simulink model "constraints_comparison_A_4D_v2"  (R2016a)
settings: Solver=ode4  StartTime=0.0  StopTime=total_time  FixedStep=0.0001  RelTol=1e-3
InitFcn:
  | % clear
  | % clc
undefined symbols (not defined in the file or in its folder): acm_aero_model, acm_T_N, breakpoints1, Cm0, Cmde, Cmq, comp_feedback, constraint_type, dail, de, dele, dele_trim, drud, Fr_mp_1, Fr_mp_2, Fr_rp_1, Fr_rp_2, ini_acm_de_deg, ini_acm_p_deg_per_s, ini_acm_phi_deg, ini_acm_psi_deg, ini_acm_q_deg_per_s, ini_acm_r_deg_per_s, ini_acm_theta_deg, ini_cmp_de_deg, ini_rig_p_deg_per_s, ini_rig_phi_deg, ini_rig_psi_deg, ini_rig_q_deg_per_s, ini_rig_r_deg_per_s, ini_rig_theta_deg, input_type, K1_svo_acm, K1_svo_cmp, K2_svo_acm, K2_svo_cmp, La, Ma, max_defl_sat_acm, max_defl_sat_cmp, max_rate_sat, max_rate_sat_acm, max_rate_sat_cmp, Na, radius, sigbuilder_block, simstop, theta_trim, thrust_trim, windspeed, Xa, Ya, Za
libraries: aerolibconvert2 x119, simulink x42, aerolibtransform2 x19, vrlib x2
(part 1 of 6)
settings Model: Creator=PD Banneheka  LastModifiedBy=PD Banneheka
settings DataIOCC: LimitDataPoints=on  SaveFormat=Array  SaveOutput=off  SaveTime=off
settings HardwareCC: ProdBitPerPointer=32  ProdLargestAtomicFloat=None  ProdIntDivRoundTo=Undefined  ProdEndianess=Unspecified  ProdWordSize=32  ProdHWDeviceType=32-bit Generic
settings ModelReferenceCC: PropagateSignalLabelsOutOfModel=off
settings ConfigComp: CovModelRefEnable=Off

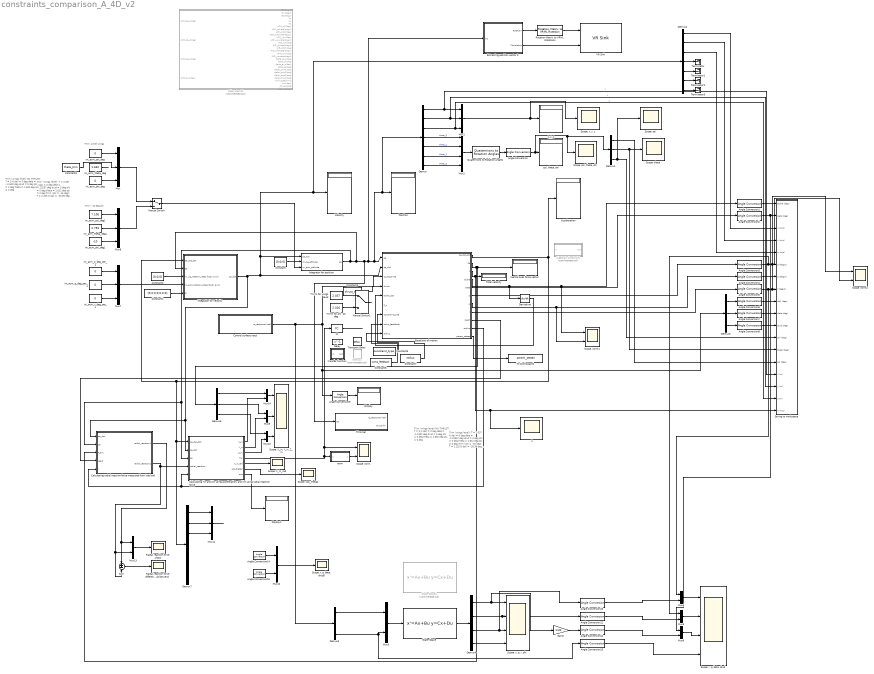
== system constraints_comparison_A_4D_v2 ==
  note: Trim: Level wings
  note: Trim (wings level):
      | T = 2.037 N
      | dail = 0 deg
      | dele = -1.22537 deg
      | drud = 0 deg
      | phi = 0 deg
      | theta = 1.612 deg
      | psi = 0 deg
      |
      | Trim (phi = -15 deg):
      | T = 2.225 N
      | dail = -30.39 deg
      | dele = -1.382 deg
      | drud = -36.89 deg
      | phi = -15.01 deg
      | theta = 5.134 deg
      | psi = 11.95 deg
      |
      | Trim (phi = -10 deg):
      | T = 2.026 N
      | dail = -18.93 deg
      | dele = -1.148 deg
      | drud = -22.97 deg
      | phi = -10 deg
      | theta = 2.793 deg
      | psi = 7.106 deg
  note: Trim (wings level):
      | T = 2.037 N
      | dail = 0 deg
      | dele = -1.22537 deg
      | drud = 0 deg
      | phi = 0 deg
      | theta = 1.612 deg
      | psi = 0 deg
      |
      | Trim (phi = -15 deg):
      | T = 2.225 N
      | dail = -30.39 deg
      | dele = -1.382 deg
      | drud = -36.89 deg
      | phi = -15.01 deg
      | theta = 5.134 deg
      | psi = 11.95 deg
      |
      | Trim (phi = -10 deg):
      | T = 2.026 N
      | dail = -18.93 deg
      | dele = -1.148 deg
      | drud = -22.97 deg
      | phi = -10 deg
      | theta = 2.793 deg
      | psi = 7.106 deg
  note: Trim: -10 deg phi
  note: Trim (wings level)
      | NO THRUST:
      | T = 0 N
      | dail = 0 deg
      | dele = -1.2402 deg
      | drud = 0 deg
      | phi = 0 deg
      | theta = 1.632 deg
      | psi = 0 deg
  note: Trim (wings level)
      | NO THRUST:
      | T = 0 N
      | dail = 0 deg
      | dele = -1.2402 deg
      | drud = 0 deg
      | phi = 0 deg
      | theta = 1.632 deg
      | psi = 0 deg
  Acceleration : Display
  Algebraic Constraint : Subsystem  Commented=on
  Angle Conversion{,1..15} (16 alike) : aerolibconvert2/Angle Conversion  IU=rad  OU=deg
  "Calculating Yin and Zin using acceleration, and Xin using radial reaction force" : MATLAB Function  TreatAsAtomicUnit=on
      settings: MinAlgLoopOccurrences=on
  Calculating radial reaction force measured from load cell : MATLAB Function  TreatAsAtomicUnit=on
      settings: MinAlgLoopOccurrences=on
  Constant : Constant  Value=[0;0;0]
  Constant1 : Constant  Value=[0;0;0;0;0;0;0]
  Constant2 : Constant  Value=[0;0;0]
  Constant3 : Constant  Value=theta_trim
  Constant4 : Constant  Value=thrust_trim
  Constant5 : Constant  Value=constraint_type
  Constant6 : Constant  Value=comp_feedback
  Constant7 : Constant  Value=radius
  Control surface input : Subsystem
  Delay : Delay  DelayLength=1  InitialCondition=0
  Demux : Demux  Outputs=7
  Demux{1,3,5..6} (4 alike) : Demux  Outputs=3
  Demux2 : Demux  Outputs=7
  Demux4 : Demux
  Demux7 : Demux  Outputs=7
  Derivative : Derivative
  Display : Display
  Display1 : Display
  Equations of motion : MATLAB Function  TreatAsAtomicUnit=on
      settings: MinAlgLoopOccurrences=on
  Extracting position vector 3 : Subsystem
  Gain2 : Gain  Gain=1/30
  IC : InitialCondition  Value=0
  Inertial axes force vector : Display
  Integrator for position : Subsystem  TreatAsAtomicUnit=on
      settings: MinAlgLoopOccurrences=on
  Integrator for velocity : Subsystem  TreatAsAtomicUnit=on
      settings: MinAlgLoopOccurrences=on
  Manual Switch : ManualSwitch
  Manual Switch1 : ManualSwitch
  Memory : Memory  Commented=on
  Mux{,1,7..8,11} (5 alike) : Mux  Inputs=3
  Mux{3..6,9..10,12..14} (9 alike) : Mux  Inputs=2
  Mux2 : Mux
  Position : Display
  Quaternions to Rotation Angles : aerolibtransform2/Quaternions to Rotation Angles  rotationOrder=ZYX
  Radial reaction force check : Scope
  Radial reaction force difference (should be zero) : Scope
  Rotation Matrix to VRML Rotation4 : vrlib/Utilities/Rotation Matrix to VRML Rotation  maxzero=1e-12
  Saving to workspace : Subsystem
  "Scope: X_in, Y_in, Z_in" : Scope  NumInputPorts=3
  Scope: X_in_rad : Scope
  Scope: cos_theta2 : Scope
  Scope: norm : Scope  NumInputPorts=2
  Scope: norm1 : Scope  NumInputPorts=2
  Scope: norm2 : Scope  NumInputPorts=2
  Scope: psi : Scope
  "Scope: psi, theta, phi" : Scope
  "Scope: r, p, beta, drud" : Scope  NumInputPorts=4
  "Scope: r, p, beta, drud5" : Scope
  Scope: theta : Scope
  "Scope: v, p, r, phi" : Scope  NumInputPorts=4
  "Scope: x, y, z" : Scope
  State-Space : StateSpace  A="[-0.8650         0  -30.0000    9.8100; -9.3510   -5.8803    2.8245         0; 5.4903   -0.1244   -2.0599         0; 0    1.0000         0         0]"  B="[0    4.5016; -213.0227  266.8872; -52.0114  -10.7994; 0         0]"  C=[1 0 0 0; 0 1 0 0; 0 0 1 0; 0 0 0 1]  D=[0 0; 0 0; 0 0; 0 0]  X0=0
  State-Space1 : StateSpace  Commented=on  A="[-0.8650         0         -30    9.8100; -10.2332   -5.8603    3.1556         0; 5.9066    0.1374   -2.1857         0; 0    1.0000         0         0]"  B="[0    4.5016; 204.6649 -268.6226; 42.5275   22.6814; 0         0]"  C=[1 0 0 0; 0 1 0 0; 0 0 1 0; 0 0 0 1]  D=[0 0; 0 0; 0 0; 0 0]  X0=0
  Subsystem14 : Subsystem  Commented=on
  Sum : Sum  Inputs=+-
  T trim for phi -10 deg : Constant  Value=2.026
  T trim for wings level : Constant  Value=2.037
  Terminator{,1..3} (4 alike) : Terminator
  To Workspace1 : ToWorkspace  VariableName=param_states  SaveFormat=Timeseries  SampleTime=-1
  Total velocity : Display
  Transport Delay : TransportDelay  DelayTime=0.1
  Trimmer : Subsystem
  V : Scope
  VR Sink : vrlib/VR Sink  InstantiateOnLoad=on  SampleTime=-1  ViewEnable=on  RemoteChange=off  RemoteView=off  FieldsWritten=Aircraft_model.rotation.4.1.1.double#Aircraft_model.translation.3.1.1.double  WorldFileName=Animation.wrl  AutoView=on  VideoDimensions=[]  AllowVariableSize=off  FigureProperties="{'Position', 'Name', 'Viewpoint', 'CameraBound', 'CameraDirection', 'CameraPosition', 'CameraUpVector', 'ZoomFactor', 'Antialiasing', 'Headlight', 'Lighting', 'NavPanel', 'Sound', 'StatusBar', 'Stereo3D', 'Stereo3DCameraOffset', 'Stereo3DHIT', 'ToolBar', 'Textures', 'Transparency', 'Triad', 'Wireframe', 'NavZones', 'NavMode', 'NavSpeed', 'CaptureFileFormat', 'CaptureFileName', 'Record2DCompressMethod', 'Record2DCompressQuality', 'Record2D', 'Record2DFileName', 'Record2DFPS'; [5.0000000000000000e+00   9.2000000000000000e+01   5.7600000000000000e+02   3.5000000000000000e+02], '', 'Front view', 'on', [0.0000000000000000e+00   0.0000000000000000e+00  -1.0000000000000000e+00], [0.0000000000000000e+00   0.0000000000000000e+00   0.0000000000000000e+00], [0.0000000000000000e+00   1.0000000000000000e+00   0.0000000000000000e+00], [1.0000000000000000e+00], 'on', 'on', 'on', 'halfbar', 'on', 'on', 'off', [1.0000000149011612e-01], [0.0000000000000000e+00], 'on', 'on', 'on', 'none', 'off', 'off', 'fly', 'normal', 'tif', '%f_anim_%n.tif', 'auto', [7.5000000000000000e+01], 'off', '%f_anim_%n.avi', 'auto'}"
  Velocity : Display
  ini_acm_p_deg_per_s : Constant  Value=0
  ini_acm_phi_deg : Constant  Value=0
  ini_acm_phi_deg1 : Constant  Value=-10
  ini_acm_psi_deg : Constant  Value=0
  ini_acm_psi_deg1 : Constant  Value=7.106
  ini_acm_q_deg_per_s : Constant  Value=0
  ini_acm_r_deg_per_s : Constant  Value=0
  ini_acm_theta_deg : Constant  Value=1.632
  ini_acm_theta_deg1 : Constant  Value=2.793
  norm : MATLAB Function  TreatAsAtomicUnit=on
  "psi, theta, phi" : Display
  transfer function : Subsystem  TreatAsAtomicUnit=on
      settings: MinAlgLoopOccurrences=on
  "x, y, z" : Display
  wires:
  Manual Switch/1 -> Integrator for position/3(ini_acm_attitude)
  Mux7/1 -> Integrator for velocity/4(ini_acm_rotation_rates (body axis))
  ini_acm_psi_deg/1 -> Mux/1
  ini_acm_theta_deg/1 -> ?
  ini_acm_phi_deg/1 -> Mux/3
  ini_acm_p_deg_per_s/1 -> Mux7/1
  ini_acm_r_deg_per_s/1 -> Mux7/3
  ini_acm_q_deg_per_s/1 -> Mux7/2
  Integrator for velocity/1(qa_dot) -> Calculating radial reaction force measured from load cell/1(qa_dot), "Calculating Yin and Zin using acceleration, and Xin using radial reaction force"/2(qa_dot), Demux2/1, Velocity/1, Integrator for position/1(qa_dot), Equations of motion/2(qa_dot)
  Constant/1 -> Integrator for position/2(ini_rig_attitude)
  Constant1/1 -> Integrator for velocity/5(qr)
  Constant2/1 -> Integrator for velocity/3(ini_rig_rotation_rates (body axis))
  Demux/4 -> Mux2/1  "theta_0"
  Demux/5 -> Mux2/2  "theta_1"
  Demux/6 -> Mux2/3  "theta_2"
  Demux/7 -> Mux2/4  "theta_3"
  Demux/3 -> Saving to workspace/17(z (m)), Mux1/3  "z"
  Demux/2 -> Saving to workspace/16(y (m)), Mux1/2  "y"
  Demux/1 -> Saving to workspace/15(x (m)), Mux1/1  "x"
  Mux1/1 -> "Scope: x, y, z"/1, "x, y, z"/1
  Mux2/1 -> Quaternions to Rotation Angles/1
  Quaternions to Rotation Angles/1 -> Angle Conversion/1
  Angle Conversion/1 -> Demux1/1, "Scope: psi, theta, phi"/1, "psi, theta, phi"/1
  Equations of motion/2(Fa) -> Demux6/1, Inertial axes force vector/1, Calculating radial reaction force measured from load cell/3(F_ext)
  Equations of motion/3(V) -> V/1, Saving to workspace/18(V (m/s)), Total velocity/1
  Equations of motion/1(qa_dot_dot) -> Integrator for velocity/1(qa_dot_dot), Demux7/1, "Calculating Yin and Zin using acceleration, and Xin using radial reaction force"/1(qa_dot_dot), Acceleration/1
  Equations of motion/4(alpha) -> Derivative/1, Scope: norm1/1, Angle Conversion1/1
  Integrator for position/1(qa) -> "Calculating Yin and Zin using acceleration, and Xin using radial reaction force"/3(qa), Calculating radial reaction force measured from load cell/2(qa), Integrator for velocity/2(qa), Trimmer/1(qa), Extracting position vector 3/1(In1), Demux/1, Position/1, Equations of motion/1(qa)
  Extracting position vector 3/1(Rotation) -> Rotation Matrix to VRML Rotation4/1
  Extracting position vector 3/2(Translation) -> VR Sink/2
  Rotation Matrix to VRML Rotation4/1 -> VR Sink/1
  Manual Switch1/1 -> ?
  Angle Conversion1/1 -> Saving to workspace/1(alpha (deg))
  Equations of motion/5(beta) -> Angle Conversion2/1
  Demux2/4 -> Terminator/1
  Demux2/6 -> Terminator2/1
  Demux2/7 -> Terminator3/1
  Demux2/5 -> Terminator1/1
  Demux2/1 -> Saving to workspace/3(u (m/s))
  Demux2/2 -> Saving to workspace/4(v (m/s))
  Demux2/3 -> Saving to workspace/5(w (m/s))
  Angle Conversion3/1 -> Mux5/1, Scope: norm2/2, Saving to workspace/6(p (deg/s))
  Angle Conversion5/1 -> Mux4/1, Scope: norm2/1, Saving to workspace/8(r (deg/s))
  Angle Conversion4/1 -> Saving to workspace/7(q (deg/s))
  Equations of motion/6(p) -> Angle Conversion3/1
  Equations of motion/7(q) -> Scope: norm1/2, Angle Conversion4/1
  Equations of motion/8(r) -> Angle Conversion5/1
  Demux3/1 -> Angle Conversion6/1
  Demux3/2 -> Angle Conversion7/1
  Demux3/3 -> Angle Conversion8/1
  Control surface input/1(cs_response (rad)) -> Equations of motion/3(cs_response), Demux3/1, Angle Conversion9/1, Demux5/1
  Demux1/1 -> Saving to workspace/14(psi (deg))
  Demux1/2 -> Saving to workspace/13(theta (deg)), Scope: theta/1
  Demux1/3 -> Scope: psi/1, Saving to workspace/12(phi (deg))
  Angle Conversion6/1 -> Saving to workspace/9(dail (deg))
  Angle Conversion7/1 -> Saving to workspace/10(dele (deg))
  Angle Conversion8/1 -> Saving to workspace/11(drud (deg))
  Mux3/1 -> State-Space/1
  State-Space/1 -> Demux4/1
  Demux5/1 -> Mux3/1
  Demux5/3 -> Mux3/2, Angle Conversion13/1
  Demux4/1 -> Gain2/1, "Scope: v, p, r, phi"/1
  Demux4/2 -> Angle Conversion11/1, "Scope: v, p, r, phi"/2
  Demux4/3 -> Angle Conversion10/1, "Scope: v, p, r, phi"/3
  Demux4/4 -> "Scope: v, p, r, phi"/4
  Gain2/1 -> Angle Conversion12/1
  Angle Conversion10/1 -> Mux4/2
  Angle Conversion11/1 -> Mux5/2
  Angle Conversion12/1 -> Mux6/2
  Mux4/1 -> "Scope: r, p, beta, drud"/1
  Mux5/1 -> "Scope: r, p, beta, drud"/2
  Mux6/1 -> "Scope: r, p, beta, drud"/3
  Angle Conversion13/1 -> "Scope: r, p, beta, drud"/4
  Angle Conversion2/1 -> Mux6/1, Saving to workspace/2(beta (deg))
  Angle Conversion9/1 -> Display/1
  Mux/1 -> Manual Switch/1
  ini_acm_psi_deg1/1 -> Mux8/1
  ini_acm_theta_deg1/1 -> Mux8/2
  ini_acm_phi_deg1/1 -> Mux8/3
  Mux8/1 -> Manual Switch/2
  T trim for wings level/1 -> Manual Switch1/1
  T trim for phi -10 deg/1 -> Manual Switch1/2
  "Calculating Yin and Zin using acceleration, and Xin using radial reaction force"/3(Z_in) -> Mux10/2
  "Calculating Yin and Zin using acceleration, and Xin using radial reaction force"/2(Y_in) -> Mux9/2
  Demux6/2 -> Mux9/1
  Demux6/3 -> Mux10/1
  Mux9/1 -> "Scope: X_in, Y_in, Z_in"/2
  Mux10/1 -> "Scope: X_in, Y_in, Z_in"/3
  Demux7/3 -> Mux11/3
  Demux7/2 -> Mux11/2
  Demux7/1 -> Mux11/1
  Mux11/1 -> ?
  Angle Conversion14/1 -> Mux12/1
  Angle Conversion15/1 -> Mux12/2
  Mux12/1 -> "Scope: r, p, beta, drud5"/1
  Equations of motion/9(react) -> Calculating radial reaction force measured from load cell/4(react)
  Calculating radial reaction force measured from load cell/1(radial_reaction1) -> Sum/1, Mux13/1
  Calculating radial reaction force measured from load cell/2(radial_reaction2) -> Sum/2, Mux13/2, "Calculating Yin and Zin using acceleration, and Xin using radial reaction force"/4(radial_reaction)
  Mux13/1 -> Radial reaction force check/1
  Sum/1 -> Radial reaction force difference (should be zero)/1
  Mux14/1 -> "Scope: X_in, Y_in, Z_in"/1
  Demux6/1 -> Mux14/1
  "Calculating Yin and Zin using acceleration, and Xin using radial reaction force"/1(X_in) -> Mux14/2
  Equations of motion/10(radius) -> Calculating radial reaction force measured from load cell/5(r), "Calculating Yin and Zin using acceleration, and Xin using radial reaction force"/5(r)
  "Calculating Yin and Zin using acceleration, and Xin using radial reaction force"/5(X_in_rad) -> Scope: X_in_rad/1
  "Calculating Yin and Zin using acceleration, and Xin using radial reaction force"/6(cos_theta2) -> Scope: cos_theta2/1
  "Calculating Yin and Zin using acceleration, and Xin using radial reaction force"/7(pos) -> Display1/1
  "Calculating Yin and Zin using acceleration, and Xin using radial reaction force"/4(F_c) -> norm/1(u), IC/1, Scope: norm/1
  norm/1(y) -> Scope: norm/2
  Derivative/1 -> Equations of motion/5(alpha_dot)
  Equations of motion/11(param_states) -> To Workspace1/1
  Constant3/1 -> Mux/2
  Constant4/1 -> Equations of motion/4(thrust)
  Constant5/1 -> Equations of motion/7(constraint_type)
  Constant6/1 -> Equations of motion/8(comp_feedback)
  IC/1 -> ?
  Constant7/1 -> Equations of motion/9("radius ")

== system constraints_comparison_A_4D_v2/Algebraic Constraint ==
  In : Inport
  Algebraic Constraint : simulink/Math Operations/Algebraic Constraint  z0=0.05076
  Algebraic Constraint{1,3..6} (5 alike) : simulink/Math Operations/Algebraic Constraint  z0=0
  Algebraic Constraint2 : simulink/Math Operations/Algebraic Constraint  z0=-0.05076
  Demux : Demux  Outputs=7
  Mux : Mux  Inputs=7
  Out : Outport
  wires:
  In/1 -> Demux/1
  Demux/7 -> Algebraic Constraint6/1
  Demux/1 -> Algebraic Constraint/1
  Demux/2 -> Algebraic Constraint1/1
  Demux/3 -> Algebraic Constraint2/1
  Demux/4 -> Algebraic Constraint3/1
  Demux/5 -> Algebraic Constraint4/1
  Demux/6 -> Algebraic Constraint5/1
  Algebraic Constraint6/1 -> Mux/7
  Algebraic Constraint5/1 -> Mux/6
  Algebraic Constraint4/1 -> Mux/5
  Algebraic Constraint3/1 -> Mux/4
  Algebraic Constraint2/1 -> Mux/3
  Algebraic Constraint1/1 -> Mux/2
  Algebraic Constraint/1 -> Mux/1
  Mux/1 -> Out/1

== system constraints_comparison_A_4D_v2/Control surface input ==
  1) Short period : Subsystem
  2) Phugoid : Subsystem  Commented=on
  3) Roll subsidence : Subsystem
  4) Spiral : Subsystem
  5) Dutch roll : Subsystem
  Aileron servo transfer function : TransferFcn  Denominator=[0.0025 0.08 1]
  Constant1 : Constant  Value=input_type
  Constant5 : Constant  Value=5
  Demux : Demux  Outputs=3
  Elevator servo transfer function : TransferFcn  Denominator=[0.0025 0.08 1]
  Manual Switch : ManualSwitch  CurrentSetting=0
  Manual Switch1 : ManualSwitch  CurrentSetting=0
  Manual Switch2 : ManualSwitch  CurrentSetting=0
  Multiport Switch : MultiPortSwitch  Inputs=5
  Mux : Mux  Inputs=3
  Rudder servo transfer function : TransferFcn  Denominator=[0.0025 0.08 1]
  cs_response (rad) : Outport
  wires:
  Manual Switch2/1 -> Mux/3  "drud"
  Manual Switch/1 -> Mux/1  "dail"
  Mux/1 -> cs_response (rad)/1
  1) Short period/1(cs_command (rad)) -> Multiport Switch/2
  2) Phugoid/1(cs_command (rad)) -> Multiport Switch/3
  3) Roll subsidence/1(cs_command (rad)) -> Multiport Switch/4
  4) Spiral/1(cs_command (rad)) -> Multiport Switch/5
  5) Dutch roll/1(cs_command (rad)) -> Multiport Switch/6
  Constant5/1 -> ?
  Multiport Switch/1 -> Demux/1
  Demux/1 -> Manual Switch/2, Aileron servo transfer function/1
  Demux/2 -> Manual Switch1/2, Elevator servo transfer function/1
  Demux/3 -> Manual Switch2/2, Rudder servo transfer function/1
  Manual Switch1/1 -> Mux/2  "dele"
  Aileron servo transfer function/1 -> Manual Switch/1  "dail"
  Elevator servo transfer function/1 -> Manual Switch1/1  "dele"
  Rudder servo transfer function/1 -> Manual Switch2/1  "drud"
  Constant1/1 -> Multiport Switch/1

== system constraints_comparison_A_4D_v2/Extracting position vector 3 ==
  In1 : Inport
  MATLAB Function : MATLAB Function  TreatAsAtomicUnit=on
  MATLAB Function1 : MATLAB Function  TreatAsAtomicUnit=on
  MATLAB Function6 : MATLAB Function  TreatAsAtomicUnit=on
  Rotation : Outport
  Translation : Outport  Port=2
  wires:
  MATLAB Function/1(y) -> Translation/1
  In1/1 -> MATLAB Function1/1(qa), MATLAB Function/1(u)
  MATLAB Function1/1(Aa) -> MATLAB Function6/1(A3)
  MATLAB Function6/1(A33) -> Rotation/1

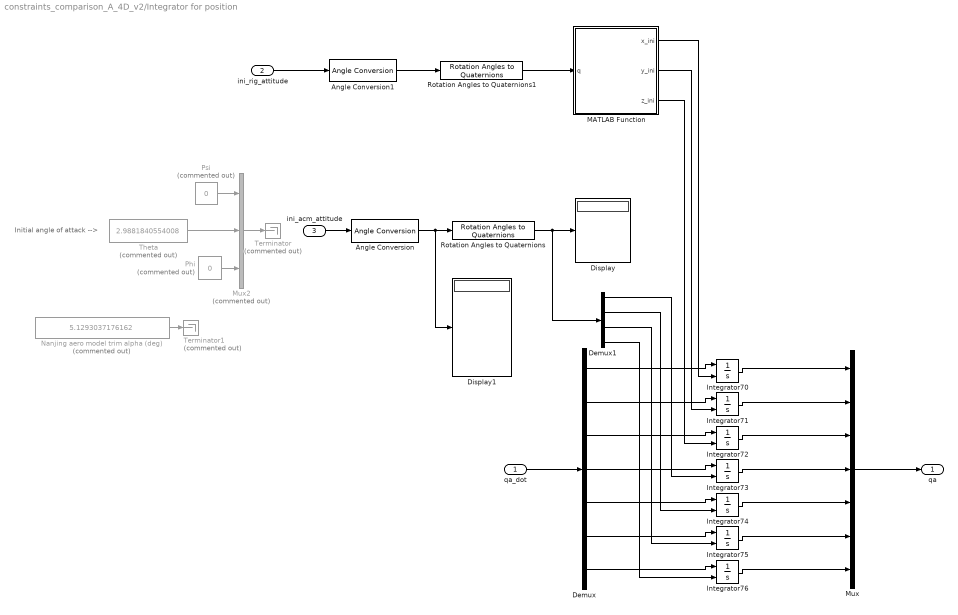
== system constraints_comparison_A_4D_v2/Integrator for position ==
  note: Initial angle of attack -->
  qa_dot : Inport
  ini_rig_attitude : Inport  Port=2
  ini_acm_attitude : Inport  Port=3
  Angle Conversion : aerolibconvert2/Angle Conversion  IU=deg  OU=rad
  Angle Conversion1 : aerolibconvert2/Angle Conversion  IU=deg  OU=rad
  Demux : Demux  Outputs=7
  Demux1 : Demux
  Display : Display
  Display1 : Display
  Integrator70 : Integrator  InitialConditionSource=external  InitialCondition=0.8
  Integrator{71..72,74..76} (5 alike) : Integrator  InitialConditionSource=external
  Integrator73 : Integrator  InitialConditionSource=external  InitialCondition=1
  MATLAB Function : MATLAB Function
  Mux : Mux  Inputs=7
  Mux2 : Mux  Commented=on  Inputs=3
  Nanjing aero model trim alpha (deg) : Constant  Commented=on  Value=5.1293037176162
  Phi : Constant  Commented=on  Value=0
  Psi : Constant  Commented=on  Value=0
  Rotation Angles to Quaternions : aerolibtransform2/Rotation Angles to Quaternions  rotationOrder=ZYX
  Rotation Angles to Quaternions1 : aerolibtransform2/Rotation Angles to Quaternions  rotationOrder=ZYX
  Terminator : Terminator  Commented=on
  Terminator1 : Terminator  Commented=on
  Theta : Constant  Commented=on  Value=2.9881840554008
  qa : Outport
  wires:
  Mux/1 -> qa/1
  qa_dot/1 -> Demux/1
  Demux/6 -> Integrator75/1
  Demux/5 -> Integrator74/1
  Demux/4 -> Integrator73/1
  Demux/3 -> Integrator72/1
  Demux/2 -> Integrator71/1
  Demux/7 -> Integrator76/1
  Demux/1 -> Integrator70/1
  Integrator76/1 -> Mux/7
  Integrator75/1 -> Mux/6
  Integrator74/1 -> Mux/5
  Integrator73/1 -> Mux/4
  Integrator72/1 -> Mux/3
  Integrator71/1 -> Mux/2
  Integrator70/1 -> Mux/1
  Phi/1 -> Mux2/3
  Psi/1 -> Mux2/1
  Mux2/1 -> Terminator/1
  Rotation Angles to Quaternions/1 -> Demux1/1, Display/1
  Demux1/4 -> Integrator76/2
  Demux1/1 -> Integrator73/2
  Demux1/2 -> Integrator74/2
  Demux1/3 -> Integrator75/2
  Angle Conversion/1 -> Display1/1, Rotation Angles to Quaternions/1
  Nanjing aero model trim alpha (deg)/1 -> Terminator1/1
  MATLAB Function/1(x_ini) -> Integrator70/2
  MATLAB Function/2(y_ini) -> Integrator71/2
  MATLAB Function/3(z_ini) -> Integrator72/2
  Theta/1 -> Mux2/2
  Angle Conversion1/1 -> Rotation Angles to Quaternions1/1
  ini_rig_attitude/1 -> Angle Conversion1/1
  ini_acm_attitude/1 -> Angle Conversion/1
  Rotation Angles to Quaternions1/1 -> MATLAB Function/1(q)

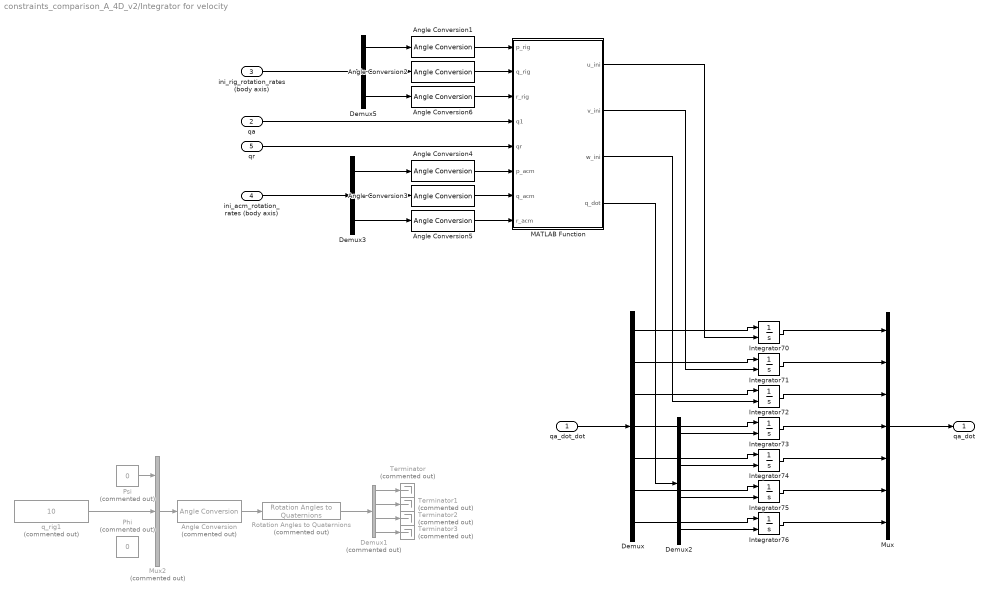
== system constraints_comparison_A_4D_v2/Integrator for velocity ==
  qa_dot_dot : Inport
  qa : Inport  Port=2
  ini_rig_rotation_rates (body axis) : Inport  Port=3
  ini_acm_rotation_rates (body axis) : Inport  Port=4
  qr : Inport  Port=5
  Angle Conversion : aerolibconvert2/Angle Conversion  Commented=on  IU=deg  OU=rad
  Angle Conversion{1..6} (6 alike) : aerolibconvert2/Angle Conversion  IU=deg  OU=rad
  Demux : Demux  Outputs=7
  Demux1 : Demux  Commented=on
  Demux2 : Demux
  Demux3 : Demux  Outputs=3
  Demux5 : Demux  Outputs=3
  Integrator{70..76} (7 alike) : Integrator  InitialConditionSource=external
  MATLAB Function : MATLAB Function
  Mux : Mux  Inputs=7
  Mux2 : Mux  Commented=on  Inputs=3
  Phi : Constant  Commented=on  Value=0
  Psi : Constant  Commented=on  Value=0
  Rotation Angles to Quaternions : aerolibtransform2/Rotation Angles to Quaternions  Commented=on  rotationOrder=ZYX
  Terminator{,1..3} (4 alike) : Terminator  Commented=on
  q_rig1 : Constant  Commented=on  Value=10
  qa_dot : Outport
  wires:
  Integrator70/1 -> Mux/1
  Integrator71/1 -> Mux/2
  Integrator72/1 -> Mux/3
  Integrator73/1 -> Mux/4
  Integrator74/1 -> Mux/5
  Integrator75/1 -> Mux/6
  Integrator76/1 -> Mux/7
  Demux/1 -> Integrator70/1
  Demux/7 -> Integrator76/1
  Demux/2 -> Integrator71/1
  Demux/3 -> Integrator72/1
  Demux/4 -> Integrator73/1
  Demux/5 -> Integrator74/1
  Demux/6 -> Integrator75/1
  qa_dot_dot/1 -> Demux/1
  Mux/1 -> qa_dot/1
  MATLAB Function/1(u_ini) -> Integrator70/2
  MATLAB Function/2(v_ini) -> Integrator71/2
  MATLAB Function/3(w_ini) -> Integrator72/2
  Angle Conversion1/1 -> MATLAB Function/1(p_rig)
  Angle Conversion2/1 -> MATLAB Function/2(q_rig)
  ini_rig_rotation_rates (body axis)/1 -> Demux5/1
  Psi/1 -> Mux2/1
  Mux2/1 -> Angle Conversion/1
  Rotation Angles to Quaternions/1 -> Demux1/1
  Angle Conversion/1 -> Rotation Angles to Quaternions/1
  q_rig1/1 -> Mux2/2
  qa/1 -> MATLAB Function/4(q1)
  Demux2/1 -> Integrator73/2
  Demux2/2 -> Integrator74/2
  Demux2/3 -> Integrator75/2
  Demux2/4 -> Integrator76/2
  MATLAB Function/4(q_dot) -> Demux2/1
  Angle Conversion3/1 -> MATLAB Function/7(q_acm)
  ini_acm_rotation_rates (body axis)/1 -> Demux3/1
  Angle Conversion4/1 -> MATLAB Function/6(p_acm)
  Angle Conversion5/1 -> MATLAB Function/8(r_acm)
  Demux3/3 -> Angle Conversion5/1
  Demux3/1 -> Angle Conversion4/1
  Demux3/2 -> Angle Conversion3/1
  Angle Conversion6/1 -> MATLAB Function/3(r_rig)
  Demux5/1 -> Angle Conversion1/1
  Demux5/2 -> Angle Conversion2/1
  Demux5/3 -> Angle Conversion6/1
  qr/1 -> MATLAB Function/5(qr)
  Demux1/2 -> Terminator1/1
  Demux1/1 -> Terminator/1
  Demux1/3 -> Terminator2/1
  Demux1/4 -> Terminator3/1

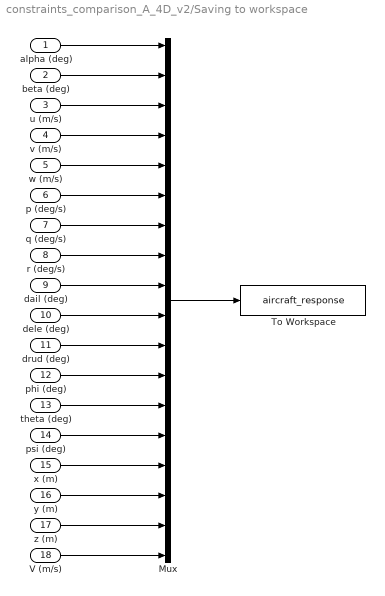
== system constraints_comparison_A_4D_v2/Saving to workspace ==
  alpha (deg) : Inport
  beta (deg) : Inport  Port=2
  u (m/s) : Inport  Port=3
  v (m/s) : Inport  Port=4
  w (m/s) : Inport  Port=5
  p (deg/s) : Inport  Port=6
  q (deg/s) : Inport  Port=7
  r (deg/s) : Inport  Port=8
  dail (deg) : Inport  Port=9
  dele (deg) : Inport  Port=10
  drud (deg) : Inport  Port=11
  phi (deg) : Inport  Port=12
  theta (deg) : Inport  Port=13
  psi (deg) : Inport  Port=14
  x (m) : Inport  Port=15
  y (m) : Inport  Port=16
  z (m) : Inport  Port=17
  V (m/s) : Inport  Port=18
  Mux : Mux  Inputs=18
  To Workspace : ToWorkspace  VariableName=aircraft_response  SaveFormat=Timeseries  SampleTime=-1
  wires:
  Mux/1 -> To Workspace/1
  alpha (deg)/1 -> Mux/1
  beta (deg)/1 -> Mux/2
  u (m/s)/1 -> Mux/3
  v (m/s)/1 -> Mux/4
  w (m/s)/1 -> Mux/5
  p (deg/s)/1 -> Mux/6
  q (deg/s)/1 -> Mux/7
  r (deg/s)/1 -> Mux/8
  dail (deg)/1 -> Mux/9
  dele (deg)/1 -> Mux/10
  drud (deg)/1 -> Mux/11
  phi (deg)/1 -> Mux/12
  theta (deg)/1 -> Mux/13
  psi (deg)/1 -> Mux/14
  z (m)/1 -> Mux/17
  V (m/s)/1 -> Mux/18
  x (m)/1 -> Mux/15
  y (m)/1 -> Mux/16
